simulink model "tests"  (R2024b)
settings: Solver=VariableStepAuto  StartTime=0.0  StopTime=1  RelTol=1e-3  AbsTol=1e-3  EnableMultiTasking=on
values from neighbouring files (symbols this model uses):
  m = obj.Br *obj.volume / obj.mu    [External_Magnet2.m]
  N = gridSizes(k)    [Test.m]
  Params = Sim_Param_Setup    [Sim_Open.m]
undefined symbols (not defined in the file or in its folder): X, Y, Z
libraries: sm_lib x88, vrlib x72, nesl_utility x52, matrix_library x46, sharedtransform x6
(part 2 of 5)

== system tests/Subsystem/Single_Arm/Plate_3 ==
  Pos_Plate6 : Inport
  M6 : Inport  Port=2
  Pos_Plate5 : Inport  Port=3
  M5 : Inport  Port=4
  Pos_Plate4 : Inport  Port=5
  M4 : Inport  Port=6
  Pos_Plate2 : Inport  Port=7
  M2 : Inport  Port=8
  Pos_Plate1 : Inport  Port=9
  M1 : Inport  Port=10
  Source_Pos : Inport  Port=11
  Source_Moment : Inport  Port=12
  Brick Solid : sm_lib/Body Elements/Brick Solid  BrickDimensions=[Params.LinkWidth Params.LinkThickness Params.LinkLength]  BrickDimensionsUnits=m  ExportEntireGeometry=off  InertiaType=CalculateFromGeometry  BasedOnType=Density  Density=1000  DensityUnits=kg/m^3  Mass=1  MassUnits=kg  CenterOfMass=[0 0 0]  CenterOfMassUnits=m  MomentsOfInertia=[1 1 1]  MomentsOfInertiaUnits=kg*m^2  ProductsOfInertia=[0 0 0]  ProductsOfInertiaUnits=kg*m^2  GraphicType=FromGeometry  MarkerShape=Sphere  MarkerSize=10  GraphicVisPropType=SimpleVisualProperties  GraphicDiffuseColor=[0.5 0.5 0.5]  GraphicOpacity=0.5  GraphicSpecularColor=[0.5 0.5 0.5 1.0]  GraphicAmbientColor=[0.15 0.15 0.15 1.0]  GraphicEmissiveColor=[0.0 0.0 0.0 1.0]  GraphicShininess=75  DoExposeReferenceFrame=on  SerializedFrames=<Frames><Frame><Id>Frame1</Id><Value><Name>F1</Name><Origin><Source>GeometricFeature</Source><FeatureName>-x -y curve</FeatureName></Origin><PrimaryAxis><DefinedDirection>+Z</DefinedDirection><Source>ReferenceFrame</Source><SourceDirection>+Z</SourceDirection><FeatureName></FeatureName></PrimaryAxis><SecondaryAxis><DefinedDirection>+X</DefinedDirection><Source>ReferenceFrame</Source><SourceDirection>+X</SourceDirection><FeatureName></FeatureName></SecondaryAxis></Value></Frame><Frame><Id>Frame2</Id><Value><Name>F2</Name><Origin><Source>GeometricFeature</Source><FeatureName>+x -y curve</FeatureName></Origin><PrimaryAxis><DefinedDirection>+Z</DefinedDirection><Source>ReferenceFrame</Source><SourceDirection>+Z</SourceDirection><FeatureName></FeatureName></PrimaryAxis><SecondaryAxis><DefinedDirection>+X</DefinedDirection><Source>ReferenceFrame</Source><SourceDirection>+X</SourceDirection><FeatureName></FeatureName></SecondaryAxis></Value></Frame></Frames>
  Constant : Constant  Value=[1; 0; 0]  VectorParams1D=off
  "Dipole Moment Angle Rot(z, theta)" : sm_lib/Frames and Transforms/Rigid Transform  RotationMethod=StandardAxis  FollAlignAxisA=+X  BaseAlignAxisA=+Y  FollAlignAxisB=+Y  BaseAlignAxisB=+Z  RotationStandardAxis=+Z  RotationAngle=Params.Link_Magnetization_Angle(3)  RotationAngleUnits=deg  RotationArbitraryAxis=[0 0 1]  RotationSequenceAxes=FollowerAxes  RotationSequence=XYX  RotationSequenceAngles=[0 0 0]  RotationSequenceAnglesUnits=deg  RotationMatrix=[1 0 0;0 1 0;0 0 1]  Quaternion=[1 0 0 0]  TranslationMethod=None  TranslationCartesianOffset=[0 0 0]  TranslationCartesianOffsetUnits=m  TranslationStandardAxis=+Z  TranslationStandardOffset=0  TranslationStandardOffsetUnits=m  TranslationROffset=0  TranslationROffsetUnits=m  TranslationThetaOffset=0  TranslationThetaOffsetUnits=deg  TranslationZOffset=0  TranslationZOffsetUnits=m
  External Force and Torque : sm_lib/Forces and Torques/External Force and Torque  EnableForceX=off  EnableForceY=off  EnableForceZ=off  EnableForce=on  ForceResolutionFrame=AttachedFrame  EnableTorqueX=off  EnableTorqueY=off  EnableTorqueZ=off  EnableTorque=on  TorqueResolutionFrame=AttachedFrame
  External Force and Torque1 : sm_lib/Forces and Torques/External Force and Torque  EnableForceX=off  EnableForceY=off  EnableForceZ=off  EnableForce=on  ForceResolutionFrame=AttachedFrame  EnableTorqueX=off  EnableTorqueY=off  EnableTorqueZ=off  EnableTorque=on  TorqueResolutionFrame=AttachedFrame
  Gain : Gain  Gain=Params.Link_Moment(3)
  PS-Simulink Converter : nesl_utility/PS-Simulink Converter  PhysicalDomain=network_engine_domain  SubClassName=ps_output  LeftPortType=input  RightPortType=output  PseudoPeriodic=off  Frequencies=[]  VectorFormat=inherit  Unit=inherit  AffineConversion=off
  PS-Simulink Converter2 : nesl_utility/PS-Simulink Converter  PhysicalDomain=network_engine_domain  SubClassName=ps_output  LeftPortType=input  RightPortType=output  PseudoPeriodic=off  Frequencies=[]  VectorFormat=inherit  Unit=inherit  AffineConversion=off
  Product : Product  Multiplication=Matrix(*)
  Revolved Solid : sm_lib/Body Elements/Revolved Solid  RevolutionCrossSection=[0 0; 1 0; 1 15; 2 15; 0 20]/10  RevolutionCrossSectionUnits=mm  RevolutionExtent=Full  RevolutionAngle=180  RevolutionAngleUnits=deg  ExportConvexHullGeometry=off  InertiaType=CalculateFromGeometry  BasedOnType=Density  Density=0  DensityUnits=kg/m^3  Mass=1  MassUnits=kg  CenterOfMass=[0 0 0]  CenterOfMassUnits=m  MomentsOfInertia=[1 1 1]  MomentsOfInertiaUnits=kg*m^2  ProductsOfInertia=[0 0 0]  ProductsOfInertiaUnits=kg*m^2  GraphicType=FromGeometry  MarkerShape=Sphere  MarkerSize=10  GraphicVisPropType=SimpleVisualProperties  GraphicDiffuseColor=[1 0 0]  GraphicOpacity=1  GraphicSpecularColor=[0.5 0.5 0.5 1.0]  GraphicAmbientColor=[0.15 0.15 0.15 1.0]  GraphicEmissiveColor=[0.0 0.0 0.0 1.0]  GraphicShininess=75  DoExposeReferenceFrame=on  SerializedFrames=<Frames/>
  Rigid Transform1 : sm_lib/Frames and Transforms/Rigid Transform  RotationMethod=StandardAxis  FollAlignAxisA=+X  BaseAlignAxisA=+Y  FollAlignAxisB=+Y  BaseAlignAxisB=+Z  RotationStandardAxis=+Y  RotationAngle=90  RotationAngleUnits=deg  RotationArbitraryAxis=[0 0 1]  RotationSequenceAxes=FollowerAxes  RotationSequence=XYX  RotationSequenceAngles=[0 0 0]  RotationSequenceAnglesUnits=deg  RotationMatrix=[1 0 0;0 1 0;0 0 1]  Quaternion=[1 0 0 0]  TranslationMethod=None  TranslationCartesianOffset=[0 0 0]  TranslationCartesianOffsetUnits=m  TranslationStandardAxis=+Z  TranslationStandardOffset=0  TranslationStandardOffsetUnits=m  TranslationROffset=0  TranslationROffsetUnits=m  TranslationThetaOffset=0  TranslationThetaOffsetUnits=deg  TranslationZOffset=0  TranslationZOffsetUnits=m
  Simulink-PS Converter{,1..3} (4 alike) : nesl_utility/Simulink-PS Converter  PhysicalDomain=network_engine_domain  SubClassName=ps_input  LeftPortType=input  RightPortType=output  PseudoPeriodic=off  Frequencies=[]  NoiseDistribution=none  NoiseParameters=[]  Unit=1  AffineConversion=off  FilteringAndDerivatives=provide  SimscapeFilterOrder=1  InputFilterTimeConstant=0.001  UdotUserProvided=0
  Subsystem : Subsystem
  Torques and Forces : Subsystem
      settings: PortSchema="{\"entries\":[{\"content\":{\"sides\":[{\"content\":{\"connectorIds\":[\"In1\",\"In2\",\"In3\",\"In4\",\"In5\",\"In6\",\"In7\",\"In8\",\"In9\",\"In10\",\"In11\",\"In12\"]},\"type\":\"ConnectorPlacement.EquallySpacedRectSide\",\"uuid\":\"5e9f7da2-fe68-4c7d-bff2-fdc8c7982441\"},{\"content\":{\"connectorIds\":[\"Out1\",\"Out2\"],\"side\":\"RIGHT\"},\"type\":\"ConnectorPlacement.EquallySpacedRectSide\",\"uuid\":\"36e5b3c2-6267-49a8-a0c4-2f3c1c270a99\"},{\"content\":{\"connectorIds\":[\"LConn1\"],\"side\":\"TOP\"},\"type\":\"ConnectorPlacement.EquallySpacedRectSide\",\"uuid\":\"f9d61316-4e06-4fe9-aa35-560b242a32a1\"}]},\"type\":\"ConnectorPlacement.EquallySpacedConnector\",\"uuid\":\"16298027-81d7-44cb-b7a6-bb815e806b74\"}],\"packageUris\":[\"http://schema.mathworks.com/mf0/Connector/R2020b\"],\"version\":\"1.0\"}"
  Transform Sensor : sm_lib/Frames and Transforms/Transform Sensor  MeasurementFrame=Base  RotationSequence=XYX  SenseAngle=off  SenseAxis=off  SenseQ=off  SenseR=on  SenseRotationSequence=off  SenseOmegaX=off  SenseOmegaY=off  SenseOmegaZ=off  SenseOmega=off  SenseQDot=off  SenseRDot=off  SenseRotationSequenceDot=off  SenseAlphaX=off  SenseAlphaY=off  SenseAlphaZ=off  SenseAlpha=off  SenseQDDot=off  SenseRDDot=off  SenseX=off  SenseY=off  SenseZ=off  SenseXYZ=on  SenseRad=off  SenseAzim=off  SenseDist=off  SenseInc=off  SenseXDot=off  SenseYDot=off  SenseZDot=off  SenseXYZDot=off  SenseRadDot=off  SenseAzimDot=off  SenseDistDot=off  SenseIncDot=off  SenseXDDot=off  SenseYDDot=off  SenseZDDot=off  SenseXYZDDot=off  SenseRadDDot=off  SenseAzimDDot=off  SenseDistDDot=off  SenseIncDDot=off
  World Frame : sm_lib/Frames and Transforms/World Frame
  Fixed one : PMIOPort  Side=Left
  base : PMIOPort  Port=2  Side=Right
  Pos_Plate3 : Outport
  M3 : Outport  Port=2
  wires:
  Gain/1 -> Product/2
  Constant/1 -> Gain/1
  Product/1 -> Torques and Forces/1(m_slave), Subsystem/1(Slave_Moment), M3/1
  PS-Simulink Converter2/1 -> Product/1
  PS-Simulink Converter/1 -> Pos_Plate3/1, Subsystem/2(Slave_Pos), Torques and Forces/2(Pos_Slave)
  M1/1 -> Torques and Forces/3(M1)
  Pos_Plate1/1 -> Torques and Forces/4(Pos_Plate1)
  M2/1 -> Torques and Forces/5(M2)
  Pos_Plate2/1 -> Torques and Forces/6(Pos_Plate2)
  M4/1 -> Torques and Forces/7(M4)
  Pos_Plate4/1 -> Torques and Forces/8(Pos_Plate4)
  M5/1 -> Torques and Forces/9(M5)
  Pos_Plate5/1 -> Torques and Forces/10(Pos_Plate5)
  M6/1 -> Torques and Forces/11(M6)
  Pos_Plate6/1 -> Torques and Forces/12(Pos_Plate6)
  Torques and Forces/1(Forces) -> Simulink-PS Converter/1
  Torques and Forces/2(Torques) -> Simulink-PS Converter1/1
  Source_Moment/1 -> Subsystem/3(Source_Moment)
  Source_Pos/1 -> Subsystem/4(Source_Pos)
  Subsystem/1(Source_Torque) -> Simulink-PS Converter3/1
  Subsystem/2(Source_Force) -> Simulink-PS Converter2/1
  connections:
  base/RConn1 -- Brick Solid/LConn1
  Brick Solid/LConn2 -- Fixed one/RConn1
  Rigid Transform1/LConn1 -- "Dipole Moment Angle Rot(z, theta)"/RConn1 -- Transform Sensor/RConn1
  Transform Sensor/RConn2 -- PS-Simulink Converter2/LConn1
  "Dipole Moment Angle Rot(z, theta)"/LConn1 -- Torques and Forces/LConn1 -- Brick Solid/RConn1 -- External Force and Torque/RConn1 -- External Force and Torque1/RConn1
  PS-Simulink Converter/LConn1 -- Transform Sensor/RConn3
  Rigid Transform1/RConn1 -- Revolved Solid/RConn1
  World Frame/RConn1 -- Transform Sensor/LConn1
  Simulink-PS Converter/RConn1 -- External Force and Torque/LConn1
  External Force and Torque/LConn2 -- Simulink-PS Converter1/RConn1
  External Force and Torque1/LConn1 -- Simulink-PS Converter2/RConn1
  Simulink-PS Converter3/RConn1 -- External Force and Torque1/LConn2

== system tests/Subsystem/Single_Arm/Plate_4 ==
  Pos_Plate6 : Inport
  M6 : Inport  Port=2
  Pos_Plate5 : Inport  Port=3
  M5 : Inport  Port=4
  Pos_Plate3 : Inport  Port=5
  M3 : Inport  Port=6
  Pos_Plate2 : Inport  Port=7
  M2 : Inport  Port=8
  Pos_Plate1 : Inport  Port=9
  M1 : Inport  Port=10
  Source_Pos : Inport  Port=11
  Source_Moment : Inport  Port=12
  Brick Solid : sm_lib/Body Elements/Brick Solid  BrickDimensions=[Params.LinkWidth Params.LinkThickness Params.LinkLength]  BrickDimensionsUnits=m  ExportEntireGeometry=off  InertiaType=CalculateFromGeometry  BasedOnType=Density  Density=1000  DensityUnits=kg/m^3  Mass=1  MassUnits=kg  CenterOfMass=[0 0 0]  CenterOfMassUnits=m  MomentsOfInertia=[1 1 1]  MomentsOfInertiaUnits=kg*m^2  ProductsOfInertia=[0 0 0]  ProductsOfInertiaUnits=kg*m^2  GraphicType=FromGeometry  MarkerShape=Sphere  MarkerSize=10  GraphicVisPropType=SimpleVisualProperties  GraphicDiffuseColor=[0.5 0.5 0.5]  GraphicOpacity=0.5  GraphicSpecularColor=[0.5 0.5 0.5 1.0]  GraphicAmbientColor=[0.15 0.15 0.15 1.0]  GraphicEmissiveColor=[0.0 0.0 0.0 1.0]  GraphicShininess=75  DoExposeReferenceFrame=on  SerializedFrames=<Frames><Frame><Id>Frame1</Id><Value><Name>F1</Name><Origin><Source>GeometricFeature</Source><FeatureName>-x -y curve</FeatureName></Origin><PrimaryAxis><DefinedDirection>+Z</DefinedDirection><Source>ReferenceFrame</Source><SourceDirection>+Z</SourceDirection><FeatureName></FeatureName></PrimaryAxis><SecondaryAxis><DefinedDirection>+X</DefinedDirection><Source>ReferenceFrame</Source><SourceDirection>+X</SourceDirection><FeatureName></FeatureName></SecondaryAxis></Value></Frame><Frame><Id>Frame2</Id><Value><Name>F2</Name><Origin><Source>GeometricFeature</Source><FeatureName>+x -y curve</FeatureName></Origin><PrimaryAxis><DefinedDirection>+Z</DefinedDirection><Source>ReferenceFrame</Source><SourceDirection>+Z</SourceDirection><FeatureName></FeatureName></PrimaryAxis><SecondaryAxis><DefinedDirection>+X</DefinedDirection><Source>ReferenceFrame</Source><SourceDirection>+X</SourceDirection><FeatureName></FeatureName></SecondaryAxis></Value></Frame></Frames>
  Constant : Constant  Value=[1; 0; 0]  VectorParams1D=off
  "Dipole Moment Angle Rot(z, theta)" : sm_lib/Frames and Transforms/Rigid Transform  RotationMethod=StandardAxis  FollAlignAxisA=+X  BaseAlignAxisA=+Y  FollAlignAxisB=+Y  BaseAlignAxisB=+Z  RotationStandardAxis=+Z  RotationAngle=Params.Link_Magnetization_Angle(4)  RotationAngleUnits=deg  RotationArbitraryAxis=[0 0 1]  RotationSequenceAxes=FollowerAxes  RotationSequence=XYX  RotationSequenceAngles=[0 0 0]  RotationSequenceAnglesUnits=deg  RotationMatrix=[1 0 0;0 1 0;0 0 1]  Quaternion=[1 0 0 0]  TranslationMethod=None  TranslationCartesianOffset=[0 0 0]  TranslationCartesianOffsetUnits=m  TranslationStandardAxis=+Z  TranslationStandardOffset=0  TranslationStandardOffsetUnits=m  TranslationROffset=0  TranslationROffsetUnits=m  TranslationThetaOffset=0  TranslationThetaOffsetUnits=deg  TranslationZOffset=0  TranslationZOffsetUnits=m
  External Force and Torque : sm_lib/Forces and Torques/External Force and Torque  EnableForceX=off  EnableForceY=off  EnableForceZ=off  EnableForce=on  ForceResolutionFrame=AttachedFrame  EnableTorqueX=off  EnableTorqueY=off  EnableTorqueZ=off  EnableTorque=on  TorqueResolutionFrame=AttachedFrame
  External Force and Torque1 : sm_lib/Forces and Torques/External Force and Torque  EnableForceX=off  EnableForceY=off  EnableForceZ=off  EnableForce=on  ForceResolutionFrame=AttachedFrame  EnableTorqueX=off  EnableTorqueY=off  EnableTorqueZ=off  EnableTorque=on  TorqueResolutionFrame=AttachedFrame
  Gain : Gain  Gain=Params.Link_Moment(4)
  PS-Simulink Converter : nesl_utility/PS-Simulink Converter  PhysicalDomain=network_engine_domain  SubClassName=ps_output  LeftPortType=input  RightPortType=output  PseudoPeriodic=off  Frequencies=[]  VectorFormat=inherit  Unit=inherit  AffineConversion=off
  PS-Simulink Converter2 : nesl_utility/PS-Simulink Converter  PhysicalDomain=network_engine_domain  SubClassName=ps_output  LeftPortType=input  RightPortType=output  PseudoPeriodic=off  Frequencies=[]  VectorFormat=inherit  Unit=inherit  AffineConversion=off
  Product : Product  Multiplication=Matrix(*)
  Revolved Solid : sm_lib/Body Elements/Revolved Solid  RevolutionCrossSection=[0 0; 1 0; 1 15; 2 15; 0 20]/10  RevolutionCrossSectionUnits=mm  RevolutionExtent=Full  RevolutionAngle=180  RevolutionAngleUnits=deg  ExportConvexHullGeometry=off  InertiaType=CalculateFromGeometry  BasedOnType=Density  Density=0  DensityUnits=kg/m^3  Mass=1  MassUnits=kg  CenterOfMass=[0 0 0]  CenterOfMassUnits=m  MomentsOfInertia=[1 1 1]  MomentsOfInertiaUnits=kg*m^2  ProductsOfInertia=[0 0 0]  ProductsOfInertiaUnits=kg*m^2  GraphicType=FromGeometry  MarkerShape=Sphere  MarkerSize=10  GraphicVisPropType=SimpleVisualProperties  GraphicDiffuseColor=[1 0 0]  GraphicOpacity=1  GraphicSpecularColor=[0.5 0.5 0.5 1.0]  GraphicAmbientColor=[0.15 0.15 0.15 1.0]  GraphicEmissiveColor=[0.0 0.0 0.0 1.0]  GraphicShininess=75  DoExposeReferenceFrame=on  SerializedFrames=<Frames/>
  Rigid Transform1 : sm_lib/Frames and Transforms/Rigid Transform  RotationMethod=StandardAxis  FollAlignAxisA=+X  BaseAlignAxisA=+Y  FollAlignAxisB=+Y  BaseAlignAxisB=+Z  RotationStandardAxis=+Y  RotationAngle=90  RotationAngleUnits=deg  RotationArbitraryAxis=[0 0 1]  RotationSequenceAxes=FollowerAxes  RotationSequence=XYX  RotationSequenceAngles=[0 0 0]  RotationSequenceAnglesUnits=deg  RotationMatrix=[1 0 0;0 1 0;0 0 1]  Quaternion=[1 0 0 0]  TranslationMethod=None  TranslationCartesianOffset=[0 0 0]  TranslationCartesianOffsetUnits=m  TranslationStandardAxis=+Z  TranslationStandardOffset=0  TranslationStandardOffsetUnits=m  TranslationROffset=0  TranslationROffsetUnits=m  TranslationThetaOffset=0  TranslationThetaOffsetUnits=deg  TranslationZOffset=0  TranslationZOffsetUnits=m
  Simulink-PS Converter{,1..3} (4 alike) : nesl_utility/Simulink-PS Converter  PhysicalDomain=network_engine_domain  SubClassName=ps_input  LeftPortType=input  RightPortType=output  PseudoPeriodic=off  Frequencies=[]  NoiseDistribution=none  NoiseParameters=[]  Unit=1  AffineConversion=off  FilteringAndDerivatives=provide  SimscapeFilterOrder=1  InputFilterTimeConstant=0.001  UdotUserProvided=0
  Subsystem : Subsystem
  Torques and Forces : Subsystem
      settings: PortSchema="{\"entries\":[{\"content\":{\"sides\":[{\"content\":{\"connectorIds\":[\"In1\",\"In2\",\"In3\",\"In4\",\"In5\",\"In6\",\"In7\",\"In8\",\"In9\",\"In10\",\"In11\",\"In12\"]},\"type\":\"ConnectorPlacement.EquallySpacedRectSide\",\"uuid\":\"5e9f7da2-fe68-4c7d-bff2-fdc8c7982441\"},{\"content\":{\"connectorIds\":[\"Out1\",\"Out2\"],\"side\":\"RIGHT\"},\"type\":\"ConnectorPlacement.EquallySpacedRectSide\",\"uuid\":\"36e5b3c2-6267-49a8-a0c4-2f3c1c270a99\"},{\"content\":{\"connectorIds\":[\"LConn1\"],\"side\":\"TOP\"},\"type\":\"ConnectorPlacement.EquallySpacedRectSide\",\"uuid\":\"f9d61316-4e06-4fe9-aa35-560b242a32a1\"}]},\"type\":\"ConnectorPlacement.EquallySpacedConnector\",\"uuid\":\"16298027-81d7-44cb-b7a6-bb815e806b74\"}],\"packageUris\":[\"http://schema.mathworks.com/mf0/Connector/R2020b\"],\"version\":\"1.0\"}"
  Transform Sensor : sm_lib/Frames and Transforms/Transform Sensor  MeasurementFrame=Base  RotationSequence=XYX  SenseAngle=off  SenseAxis=off  SenseQ=off  SenseR=on  SenseRotationSequence=off  SenseOmegaX=off  SenseOmegaY=off  SenseOmegaZ=off  SenseOmega=off  SenseQDot=off  SenseRDot=off  SenseRotationSequenceDot=off  SenseAlphaX=off  SenseAlphaY=off  SenseAlphaZ=off  SenseAlpha=off  SenseQDDot=off  SenseRDDot=off  SenseX=off  SenseY=off  SenseZ=off  SenseXYZ=on  SenseRad=off  SenseAzim=off  SenseDist=off  SenseInc=off  SenseXDot=off  SenseYDot=off  SenseZDot=off  SenseXYZDot=off  SenseRadDot=off  SenseAzimDot=off  SenseDistDot=off  SenseIncDot=off  SenseXDDot=off  SenseYDDot=off  SenseZDDot=off  SenseXYZDDot=off  SenseRadDDot=off  SenseAzimDDot=off  SenseDistDDot=off  SenseIncDDot=off
  World Frame : sm_lib/Frames and Transforms/World Frame
  Fixed one : PMIOPort  Side=Left
  base : PMIOPort  Port=2  Side=Right
  Pos_Plate4 : Outport
  M4 : Outport  Port=2
  wires:
  PS-Simulink Converter/1 -> Subsystem/2(Slave_Pos), Torques and Forces/2(Pos_Slave), Pos_Plate4/1
  Product/1 -> Torques and Forces/1(m_slave), Subsystem/1(Slave_Moment), M4/1
  Gain/1 -> Product/2
  Constant/1 -> Gain/1
  PS-Simulink Converter2/1 -> Product/1
  M1/1 -> Torques and Forces/3(M1)
  Pos_Plate1/1 -> Torques and Forces/4(Pos_Plate1)
  M2/1 -> Torques and Forces/5(M2)
  Pos_Plate2/1 -> Torques and Forces/6(Pos_Plate2)
  M3/1 -> Torques and Forces/7(M3)
  Pos_Plate3/1 -> Torques and Forces/8(Pos_Plate3)
  M5/1 -> Torques and Forces/9(M5)
  Pos_Plate5/1 -> Torques and Forces/10(Pos_Plate5)
  M6/1 -> Torques and Forces/11(M6)
  Pos_Plate6/1 -> Torques and Forces/12(Pos_Plate6)
  Torques and Forces/1(Forces) -> Simulink-PS Converter/1
  Torques and Forces/2(Torques) -> Simulink-PS Converter1/1
  Source_Moment/1 -> Subsystem/3(Source_Moment)
  Source_Pos/1 -> Subsystem/4(Source_Pos)
  Subsystem/1(Source_Torque) -> Simulink-PS Converter3/1
  Subsystem/2(Source_Force) -> Simulink-PS Converter2/1
  connections:
  base/RConn1 -- Brick Solid/LConn1
  Brick Solid/LConn2 -- Fixed one/RConn1
  Rigid Transform1/LConn1 -- "Dipole Moment Angle Rot(z, theta)"/RConn1 -- Transform Sensor/RConn1
  World Frame/RConn1 -- Transform Sensor/LConn1
  Rigid Transform1/RConn1 -- Revolved Solid/RConn1
  PS-Simulink Converter/LConn1 -- Transform Sensor/RConn3
  Brick Solid/RConn1 -- Torques and Forces/LConn1 -- External Force and Torque/RConn1 -- External Force and Torque1/RConn1 -- "Dipole Moment Angle Rot(z, theta)"/LConn1
  Transform Sensor/RConn2 -- PS-Simulink Converter2/LConn1
  External Force and Torque/LConn2 -- Simulink-PS Converter1/RConn1
  Simulink-PS Converter/RConn1 -- External Force and Torque/LConn1
  External Force and Torque1/LConn1 -- Simulink-PS Converter2/RConn1
  Simulink-PS Converter3/RConn1 -- External Force and Torque1/LConn2

== system tests/Subsystem/Single_Arm/Plate_5 ==
  Pos_Plate6 : Inport
  M6 : Inport  Port=2
  Pos_Plate4 : Inport  Port=3
  M4 : Inport  Port=4
  Pos_Plate3 : Inport  Port=5
  M3 : Inport  Port=6
  Pos_Plate2 : Inport  Port=7
  M2 : Inport  Port=8
  Pos_Plate1 : Inport  Port=9
  M1 : Inport  Port=10
  Source_Pos : Inport  Port=11
  Source_Moment : Inport  Port=12
  Brick Solid : sm_lib/Body Elements/Brick Solid  BrickDimensions=[Params.LinkWidth Params.LinkThickness Params.LinkLength]  BrickDimensionsUnits=m  ExportEntireGeometry=off  InertiaType=CalculateFromGeometry  BasedOnType=Density  Density=1000  DensityUnits=kg/m^3  Mass=1  MassUnits=kg  CenterOfMass=[0 0 0]  CenterOfMassUnits=m  MomentsOfInertia=[1 1 1]  MomentsOfInertiaUnits=kg*m^2  ProductsOfInertia=[0 0 0]  ProductsOfInertiaUnits=kg*m^2  GraphicType=FromGeometry  MarkerShape=Sphere  MarkerSize=10  GraphicVisPropType=SimpleVisualProperties  GraphicDiffuseColor=[0.5 0.5 0.5]  GraphicOpacity=0.5  GraphicSpecularColor=[0.5 0.5 0.5 1.0]  GraphicAmbientColor=[0.15 0.15 0.15 1.0]  GraphicEmissiveColor=[0.0 0.0 0.0 1.0]  GraphicShininess=75  DoExposeReferenceFrame=on  SerializedFrames=<Frames><Frame><Id>Frame1</Id><Value><Name>F1</Name><Origin><Source>GeometricFeature</Source><FeatureName>-x -y curve</FeatureName></Origin><PrimaryAxis><DefinedDirection>+Z</DefinedDirection><Source>ReferenceFrame</Source><SourceDirection>+Z</SourceDirection><FeatureName></FeatureName></PrimaryAxis><SecondaryAxis><DefinedDirection>+X</DefinedDirection><Source>ReferenceFrame</Source><SourceDirection>+X</SourceDirection><FeatureName></FeatureName></SecondaryAxis></Value></Frame><Frame><Id>Frame2</Id><Value><Name>F2</Name><Origin><Source>GeometricFeature</Source><FeatureName>+x -y curve</FeatureName></Origin><PrimaryAxis><DefinedDirection>+Z</DefinedDirection><Source>ReferenceFrame</Source><SourceDirection>+Z</SourceDirection><FeatureName></FeatureName></PrimaryAxis><SecondaryAxis><DefinedDirection>+X</DefinedDirection><Source>ReferenceFrame</Source><SourceDirection>+X</SourceDirection><FeatureName></FeatureName></SecondaryAxis></Value></Frame></Frames>
  Constant : Constant  Value=[1; 0; 0]  VectorParams1D=off
  "Dipole Moment Angle Rot(z, theta)" : sm_lib/Frames and Transforms/Rigid Transform  RotationMethod=StandardAxis  FollAlignAxisA=+X  BaseAlignAxisA=+Y  FollAlignAxisB=+Y  BaseAlignAxisB=+Z  RotationStandardAxis=+Z  RotationAngle=Params.Link_Magnetization_Angle(5)  RotationAngleUnits=deg  RotationArbitraryAxis=[0 0 1]  RotationSequenceAxes=FollowerAxes  RotationSequence=XYX  RotationSequenceAngles=[0 0 0]  RotationSequenceAnglesUnits=deg  RotationMatrix=[1 0 0;0 1 0;0 0 1]  Quaternion=[1 0 0 0]  TranslationMethod=None  TranslationCartesianOffset=[0 0 0]  TranslationCartesianOffsetUnits=m  TranslationStandardAxis=+Z  TranslationStandardOffset=0  TranslationStandardOffsetUnits=m  TranslationROffset=0  TranslationROffsetUnits=m  TranslationThetaOffset=0  TranslationThetaOffsetUnits=deg  TranslationZOffset=0  TranslationZOffsetUnits=m
  External Force and Torque : sm_lib/Forces and Torques/External Force and Torque  EnableForceX=off  EnableForceY=off  EnableForceZ=off  EnableForce=on  ForceResolutionFrame=AttachedFrame  EnableTorqueX=off  EnableTorqueY=off  EnableTorqueZ=off  EnableTorque=on  TorqueResolutionFrame=AttachedFrame
  External Force and Torque1 : sm_lib/Forces and Torques/External Force and Torque  EnableForceX=off  EnableForceY=off  EnableForceZ=off  EnableForce=on  ForceResolutionFrame=AttachedFrame  EnableTorqueX=off  EnableTorqueY=off  EnableTorqueZ=off  EnableTorque=on  TorqueResolutionFrame=AttachedFrame
  Gain : Gain  Gain=Params.Link_Moment(5)
  PS-Simulink Converter : nesl_utility/PS-Simulink Converter  PhysicalDomain=network_engine_domain  SubClassName=ps_output  LeftPortType=input  RightPortType=output  PseudoPeriodic=off  Frequencies=[]  VectorFormat=inherit  Unit=inherit  AffineConversion=off
  PS-Simulink Converter2 : nesl_utility/PS-Simulink Converter  PhysicalDomain=network_engine_domain  SubClassName=ps_output  LeftPortType=input  RightPortType=output  PseudoPeriodic=off  Frequencies=[]  VectorFormat=inherit  Unit=inherit  AffineConversion=off
  Product : Product  Multiplication=Matrix(*)
  Revolved Solid : sm_lib/Body Elements/Revolved Solid  RevolutionCrossSection=[0 0; 1 0; 1 15; 2 15; 0 20]/10  RevolutionCrossSectionUnits=mm  RevolutionExtent=Full  RevolutionAngle=180  RevolutionAngleUnits=deg  ExportConvexHullGeometry=off  InertiaType=CalculateFromGeometry  BasedOnType=Density  Density=0  DensityUnits=kg/m^3  Mass=1  MassUnits=kg  CenterOfMass=[0 0 0]  CenterOfMassUnits=m  MomentsOfInertia=[1 1 1]  MomentsOfInertiaUnits=kg*m^2  ProductsOfInertia=[0 0 0]  ProductsOfInertiaUnits=kg*m^2  GraphicType=FromGeometry  MarkerShape=Sphere  MarkerSize=10  GraphicVisPropType=SimpleVisualProperties  GraphicDiffuseColor=[1 0 0]  GraphicOpacity=1  GraphicSpecularColor=[0.5 0.5 0.5 1.0]  GraphicAmbientColor=[0.15 0.15 0.15 1.0]  GraphicEmissiveColor=[0.0 0.0 0.0 1.0]  GraphicShininess=75  DoExposeReferenceFrame=on  SerializedFrames=<Frames/>
  Rigid Transform1 : sm_lib/Frames and Transforms/Rigid Transform  RotationMethod=StandardAxis  FollAlignAxisA=+X  BaseAlignAxisA=+Y  FollAlignAxisB=+Y  BaseAlignAxisB=+Z  RotationStandardAxis=+Y  RotationAngle=90  RotationAngleUnits=deg  RotationArbitraryAxis=[0 0 1]  RotationSequenceAxes=FollowerAxes  RotationSequence=XYX  RotationSequenceAngles=[0 0 0]  RotationSequenceAnglesUnits=deg  RotationMatrix=[1 0 0;0 1 0;0 0 1]  Quaternion=[1 0 0 0]  TranslationMethod=None  TranslationCartesianOffset=[0 0 0]  TranslationCartesianOffsetUnits=m  TranslationStandardAxis=+Z  TranslationStandardOffset=0  TranslationStandardOffsetUnits=m  TranslationROffset=0  TranslationROffsetUnits=m  TranslationThetaOffset=0  TranslationThetaOffsetUnits=deg  TranslationZOffset=0  TranslationZOffsetUnits=m
  Simulink-PS Converter{,1..3} (4 alike) : nesl_utility/Simulink-PS Converter  PhysicalDomain=network_engine_domain  SubClassName=ps_input  LeftPortType=input  RightPortType=output  PseudoPeriodic=off  Frequencies=[]  NoiseDistribution=none  NoiseParameters=[]  Unit=1  AffineConversion=off  FilteringAndDerivatives=provide  SimscapeFilterOrder=1  InputFilterTimeConstant=0.001  UdotUserProvided=0
  Subsystem : Subsystem
  Torques and Forces : Subsystem
      settings: PortSchema="{\"entries\":[{\"content\":{\"sides\":[{\"content\":{\"connectorIds\":[\"In1\",\"In2\",\"In3\",\"In4\",\"In5\",\"In6\",\"In7\",\"In8\",\"In9\",\"In10\",\"In11\",\"In12\"]},\"type\":\"ConnectorPlacement.EquallySpacedRectSide\",\"uuid\":\"5e9f7da2-fe68-4c7d-bff2-fdc8c7982441\"},{\"content\":{\"connectorIds\":[\"Out1\",\"Out2\"],\"side\":\"RIGHT\"},\"type\":\"ConnectorPlacement.EquallySpacedRectSide\",\"uuid\":\"36e5b3c2-6267-49a8-a0c4-2f3c1c270a99\"},{\"content\":{\"connectorIds\":[\"LConn1\"],\"side\":\"TOP\"},\"type\":\"ConnectorPlacement.EquallySpacedRectSide\",\"uuid\":\"f9d61316-4e06-4fe9-aa35-560b242a32a1\"}]},\"type\":\"ConnectorPlacement.EquallySpacedConnector\",\"uuid\":\"16298027-81d7-44cb-b7a6-bb815e806b74\"}],\"packageUris\":[\"http://schema.mathworks.com/mf0/Connector/R2020b\"],\"version\":\"1.0\"}"
  Transform Sensor : sm_lib/Frames and Transforms/Transform Sensor  MeasurementFrame=Base  RotationSequence=XYX  SenseAngle=off  SenseAxis=off  SenseQ=off  SenseR=on  SenseRotationSequence=off  SenseOmegaX=off  SenseOmegaY=off  SenseOmegaZ=off  SenseOmega=off  SenseQDot=off  SenseRDot=off  SenseRotationSequenceDot=off  SenseAlphaX=off  SenseAlphaY=off  SenseAlphaZ=off  SenseAlpha=off  SenseQDDot=off  SenseRDDot=off  SenseX=off  SenseY=off  SenseZ=off  SenseXYZ=on  SenseRad=off  SenseAzim=off  SenseDist=off  SenseInc=off  SenseXDot=off  SenseYDot=off  SenseZDot=off  SenseXYZDot=off  SenseRadDot=off  SenseAzimDot=off  SenseDistDot=off  SenseIncDot=off  SenseXDDot=off  SenseYDDot=off  SenseZDDot=off  SenseXYZDDot=off  SenseRadDDot=off  SenseAzimDDot=off  SenseDistDDot=off  SenseIncDDot=off
  World Frame : sm_lib/Frames and Transforms/World Frame
  Fixed one : PMIOPort  Side=Left
  base : PMIOPort  Port=2  Side=Right
  Pos_Plate5 : Outport
  M5 : Outport  Port=2
  wires:
  PS-Simulink Converter/1 -> Subsystem/2(Slave_Pos), Torques and Forces/2(Pos_Slave), Pos_Plate5/1
  Product/1 -> Torques and Forces/1(m_slave), Subsystem/1(Slave_Moment), M5/1
  Gain/1 -> Product/2
  Constant/1 -> Gain/1
  PS-Simulink Converter2/1 -> Product/1
  M1/1 -> Torques and Forces/3(M1)
  Pos_Plate1/1 -> Torques and Forces/4(Pos_Plate1)
  M2/1 -> Torques and Forces/5(M2)
  Pos_Plate2/1 -> Torques and Forces/6(Pos_Plate2)
  M3/1 -> Torques and Forces/7(M3)
  Pos_Plate3/1 -> Torques and Forces/8(Pos_Plate3)
  M4/1 -> Torques and Forces/9(M4)
  Pos_Plate4/1 -> Torques and Forces/10(Pos_Plate4)
  M6/1 -> Torques and Forces/11(M6)
  Pos_Plate6/1 -> Torques and Forces/12(Pos_Plate6)
  Torques and Forces/1(Forces) -> Simulink-PS Converter/1
  Torques and Forces/2(Torques) -> Simulink-PS Converter1/1
  Source_Moment/1 -> Subsystem/3(Source_Moment)
  Source_Pos/1 -> Subsystem/4(Source_Pos)
  Subsystem/1(Source_Torque) -> Simulink-PS Converter3/1
  Subsystem/2(Source_Force) -> Simulink-PS Converter2/1
  connections:
  base/RConn1 -- Brick Solid/LConn1
  Brick Solid/LConn2 -- Fixed one/RConn1
  Rigid Transform1/LConn1 -- "Dipole Moment Angle Rot(z, theta)"/RConn1 -- Transform Sensor/RConn1
  World Frame/RConn1 -- Transform Sensor/LConn1
  Rigid Transform1/RConn1 -- Revolved Solid/RConn1
  PS-Simulink Converter/LConn1 -- Transform Sensor/RConn3
  Brick Solid/RConn1 -- External Force and Torque1/RConn1 -- "Dipole Moment Angle Rot(z, theta)"/LConn1 -- External Force and Torque/RConn1 -- Torques and Forces/LConn1
  Transform Sensor/RConn2 -- PS-Simulink Converter2/LConn1
  External Force and Torque/LConn2 -- Simulink-PS Converter1/RConn1
  Simulink-PS Converter/RConn1 -- External Force and Torque/LConn1
  External Force and Torque1/LConn1 -- Simulink-PS Converter2/RConn1
  Simulink-PS Converter3/RConn1 -- External Force and Torque1/LConn2

== system tests/Subsystem/Single_Arm/Plate_6 ==
  Pos_Plate5 : Inport
  M5 : Inport  Port=2
  Pos_Plate4 : Inport  Port=3
  M4 : Inport  Port=4
  Pos_Plate3 : Inport  Port=5
  M3 : Inport  Port=6
  Pos_Plate2 : Inport  Port=7
  M2 : Inport  Port=8
  Pos_Plate1 : Inport  Port=9
  M1 : Inport  Port=10
  Source_Pos : Inport  Port=11
  Source_Moment : Inport  Port=12
  Brick Solid : sm_lib/Body Elements/Brick Solid  BrickDimensions=[Params.LinkWidth Params.LinkThickness Params.LinkLength]  BrickDimensionsUnits=m  ExportEntireGeometry=off  InertiaType=CalculateFromGeometry  BasedOnType=Density  Density=1000  DensityUnits=kg/m^3  Mass=1  MassUnits=kg  CenterOfMass=[0 0 0]  CenterOfMassUnits=m  MomentsOfInertia=[1 1 1]  MomentsOfInertiaUnits=kg*m^2  ProductsOfInertia=[0 0 0]  ProductsOfInertiaUnits=kg*m^2  GraphicType=FromGeometry  MarkerShape=Sphere  MarkerSize=10  GraphicVisPropType=SimpleVisualProperties  GraphicDiffuseColor=[0.5 0.5 0.5]  GraphicOpacity=0.5  GraphicSpecularColor=[0.5 0.5 0.5 1.0]  GraphicAmbientColor=[0.15 0.15 0.15 1.0]  GraphicEmissiveColor=[0.0 0.0 0.0 1.0]  GraphicShininess=75  DoExposeReferenceFrame=on  SerializedFrames=<Frames><Frame><Id>Frame1</Id><Value><Name>F1</Name><Origin><Source>GeometricFeature</Source><FeatureName>-x -y curve</FeatureName></Origin><PrimaryAxis><DefinedDirection>+Z</DefinedDirection><Source>ReferenceFrame</Source><SourceDirection>+Z</SourceDirection><FeatureName></FeatureName></PrimaryAxis><SecondaryAxis><DefinedDirection>+X</DefinedDirection><Source>ReferenceFrame</Source><SourceDirection>+X</SourceDirection><FeatureName></FeatureName></SecondaryAxis></Value></Frame><Frame><Id>Frame2</Id><Value><Name>F2</Name><Origin><Source>GeometricFeature</Source><FeatureName>+x -y curve</FeatureName></Origin><PrimaryAxis><DefinedDirection>+Z</DefinedDirection><Source>ReferenceFrame</Source><SourceDirection>+Z</SourceDirection><FeatureName></FeatureName></PrimaryAxis><SecondaryAxis><DefinedDirection>+X</DefinedDirection><Source>ReferenceFrame</Source><SourceDirection>+X</SourceDirection><FeatureName></FeatureName></SecondaryAxis></Value></Frame></Frames>
  Constant : Constant  Value=[1; 0; 0]  VectorParams1D=off
  "Dipole Moment Angle Rot(z, theta)" : sm_lib/Frames and Transforms/Rigid Transform  RotationMethod=StandardAxis  FollAlignAxisA=+X  BaseAlignAxisA=+Y  FollAlignAxisB=+Y  BaseAlignAxisB=+Z  RotationStandardAxis=+Z  RotationAngle=Params.Link_Magnetization_Angle(6)  RotationAngleUnits=deg  RotationArbitraryAxis=[0 0 1]  RotationSequenceAxes=FollowerAxes  RotationSequence=XYX  RotationSequenceAngles=[0 0 0]  RotationSequenceAnglesUnits=deg  RotationMatrix=[1 0 0;0 1 0;0 0 1]  Quaternion=[1 0 0 0]  TranslationMethod=None  TranslationCartesianOffset=[0 0 0]  TranslationCartesianOffsetUnits=m  TranslationStandardAxis=+Z  TranslationStandardOffset=0  TranslationStandardOffsetUnits=m  TranslationROffset=0  TranslationROffsetUnits=m  TranslationThetaOffset=0  TranslationThetaOffsetUnits=deg  TranslationZOffset=0  TranslationZOffsetUnits=m
  External Force and Torque : sm_lib/Forces and Torques/External Force and Torque  EnableForceX=off  EnableForceY=off  EnableForceZ=off  EnableForce=on  ForceResolutionFrame=AttachedFrame  EnableTorqueX=off  EnableTorqueY=off  EnableTorqueZ=off  EnableTorque=on  TorqueResolutionFrame=AttachedFrame
  External Force and Torque1 : sm_lib/Forces and Torques/External Force and Torque  EnableForceX=off  EnableForceY=off  EnableForceZ=off  EnableForce=on  ForceResolutionFrame=AttachedFrame  EnableTorqueX=off  EnableTorqueY=off  EnableTorqueZ=off  EnableTorque=on  TorqueResolutionFrame=AttachedFrame
  Gain : Gain  Gain=Params.Link_Moment(6)
  PS-Simulink Converter : nesl_utility/PS-Simulink Converter  PhysicalDomain=network_engine_domain  SubClassName=ps_output  LeftPortType=input  RightPortType=output  PseudoPeriodic=off  Frequencies=[]  VectorFormat=inherit  Unit=inherit  AffineConversion=off
  PS-Simulink Converter2 : nesl_utility/PS-Simulink Converter  PhysicalDomain=network_engine_domain  SubClassName=ps_output  LeftPortType=input  RightPortType=output  PseudoPeriodic=off  Frequencies=[]  VectorFormat=inherit  Unit=inherit  AffineConversion=off
  Product : Product  Multiplication=Matrix(*)
  Revolved Solid : sm_lib/Body Elements/Revolved Solid  RevolutionCrossSection=[0 0; 1 0; 1 15; 2 15; 0 20]/10  RevolutionCrossSectionUnits=mm  RevolutionExtent=Full  RevolutionAngle=180  RevolutionAngleUnits=deg  ExportConvexHullGeometry=off  InertiaType=CalculateFromGeometry  BasedOnType=Density  Density=0  DensityUnits=kg/m^3  Mass=1  MassUnits=kg  CenterOfMass=[0 0 0]  CenterOfMassUnits=m  MomentsOfInertia=[1 1 1]  MomentsOfInertiaUnits=kg*m^2  ProductsOfInertia=[0 0 0]  ProductsOfInertiaUnits=kg*m^2  GraphicType=FromGeometry  MarkerShape=Sphere  MarkerSize=10  GraphicVisPropType=SimpleVisualProperties  GraphicDiffuseColor=[1 0 0]  GraphicOpacity=1  GraphicSpecularColor=[0.5 0.5 0.5 1.0]  GraphicAmbientColor=[0.15 0.15 0.15 1.0]  GraphicEmissiveColor=[0.0 0.0 0.0 1.0]  GraphicShininess=75  DoExposeReferenceFrame=on  SerializedFrames=<Frames/>
  Rigid Transform1 : sm_lib/Frames and Transforms/Rigid Transform  RotationMethod=StandardAxis  FollAlignAxisA=+X  BaseAlignAxisA=+Y  FollAlignAxisB=+Y  BaseAlignAxisB=+Z  RotationStandardAxis=+Y  RotationAngle=90  RotationAngleUnits=deg  RotationArbitraryAxis=[0 0 1]  RotationSequenceAxes=FollowerAxes  RotationSequence=XYX  RotationSequenceAngles=[0 0 0]  RotationSequenceAnglesUnits=deg  RotationMatrix=[1 0 0;0 1 0;0 0 1]  Quaternion=[1 0 0 0]  TranslationMethod=None  TranslationCartesianOffset=[0 0 0]  TranslationCartesianOffsetUnits=m  TranslationStandardAxis=+Z  TranslationStandardOffset=0  TranslationStandardOffsetUnits=m  TranslationROffset=0  TranslationROffsetUnits=m  TranslationThetaOffset=0  TranslationThetaOffsetUnits=deg  TranslationZOffset=0  TranslationZOffsetUnits=m
  Simulink-PS Converter{,1..3} (4 alike) : nesl_utility/Simulink-PS Converter  PhysicalDomain=network_engine_domain  SubClassName=ps_input  LeftPortType=input  RightPortType=output  PseudoPeriodic=off  Frequencies=[]  NoiseDistribution=none  NoiseParameters=[]  Unit=1  AffineConversion=off  FilteringAndDerivatives=provide  SimscapeFilterOrder=1  InputFilterTimeConstant=0.001  UdotUserProvided=0
  Subsystem : Subsystem
  Torques and Forces : Subsystem
      settings: PortSchema="{\"entries\":[{\"content\":{\"sides\":[{\"content\":{\"connectorIds\":[\"In1\",\"In2\",\"In3\",\"In4\",\"In5\",\"In6\",\"In7\",\"In8\",\"In9\",\"In10\",\"In11\",\"In12\"]},\"type\":\"ConnectorPlacement.EquallySpacedRectSide\",\"uuid\":\"ff28c452-50a3-45d4-b830-c141bf0d4924\"},{\"content\":{\"connectorIds\":[\"Out1\",\"Out2\"],\"side\":\"RIGHT\"},\"type\":\"ConnectorPlacement.EquallySpacedRectSide\",\"uuid\":\"4d65d73f-a147-470a-914d-b752947974df\"},{\"content\":{\"connectorIds\":[\"LConn1\"],\"side\":\"TOP\"},\"type\":\"ConnectorPlacement.EquallySpacedRectSide\",\"uuid\":\"638f3315-7fa0-4e2a-8069-7601753d6a25\"}]},\"type\":\"ConnectorPlacement.EquallySpacedConnector\",\"uuid\":\"2ec04731-f5c0-4183-a2fa-470eff73c2d9\"}],\"packageUris\":[\"http://schema.mathworks.com/mf0/Connector/R2020b\"],\"version\":\"1.0\"}"
  Transform Sensor : sm_lib/Frames and Transforms/Transform Sensor  MeasurementFrame=Base  RotationSequence=XYX  SenseAngle=off  SenseAxis=off  SenseQ=off  SenseR=on  SenseRotationSequence=off  SenseOmegaX=off  SenseOmegaY=off  SenseOmegaZ=off  SenseOmega=off  SenseQDot=off  SenseRDot=off  SenseRotationSequenceDot=off  SenseAlphaX=off  SenseAlphaY=off  SenseAlphaZ=off  SenseAlpha=off  SenseQDDot=off  SenseRDDot=off  SenseX=off  SenseY=off  SenseZ=off  SenseXYZ=on  SenseRad=off  SenseAzim=off  SenseDist=off  SenseInc=off  SenseXDot=off  SenseYDot=off  SenseZDot=off  SenseXYZDot=off  SenseRadDot=off  SenseAzimDot=off  SenseDistDot=off  SenseIncDot=off  SenseXDDot=off  SenseYDDot=off  SenseZDDot=off  SenseXYZDDot=off  SenseRadDDot=off  SenseAzimDDot=off  SenseDistDDot=off  SenseIncDDot=off
  World Frame : sm_lib/Frames and Transforms/World Frame
  Fixed one : PMIOPort  Side=Left
  base : PMIOPort  Port=2  Side=Right
  Pos_Plate6 : Outport
  M6 : Outport  Port=2
  wires:
  PS-Simulink Converter/1 -> Torques and Forces/2(Pos_Slave), Pos_Plate6/1, Subsystem/2(Slave_Pos)
  Product/1 -> Subsystem/1(Slave_Moment), Torques and Forces/1(m_slave), M6/1
  Gain/1 -> Product/2
  Constant/1 -> Gain/1
  PS-Simulink Converter2/1 -> Product/1
  M1/1 -> Torques and Forces/3(M1)
  Pos_Plate1/1 -> Torques and Forces/4(Pos_Plate1)
  M2/1 -> Torques and Forces/5(M2)
  Pos_Plate2/1 -> Torques and Forces/6(Pos_Plate2)
  M3/1 -> Torques and Forces/7(M3)
  Pos_Plate3/1 -> Torques and Forces/8(Pos_Plate3)
  M4/1 -> Torques and Forces/9(M4)
  Pos_Plate4/1 -> Torques and Forces/10(Pos_Plate4)
  M5/1 -> Torques and Forces/11(M5)
  Pos_Plate5/1 -> Torques and Forces/12(Pos_Plate5)
  Torques and Forces/1(Forces) -> Simulink-PS Converter/1
  Torques and Forces/2(Torques) -> Simulink-PS Converter1/1
  Source_Moment/1 -> Subsystem/3(Source_Moment)
  Source_Pos/1 -> Subsystem/4(Source_Pos)
  Subsystem/1(Source_Torque) -> Simulink-PS Converter3/1
  Subsystem/2(Source_Force) -> Simulink-PS Converter2/1
  connections:
  base/RConn1 -- Brick Solid/LConn1
  Brick Solid/LConn2 -- Fixed one/RConn1
  Rigid Transform1/LConn1 -- "Dipole Moment Angle Rot(z, theta)"/RConn1 -- Transform Sensor/RConn1
  World Frame/RConn1 -- Transform Sensor/LConn1
  Rigid Transform1/RConn1 -- Revolved Solid/RConn1
  PS-Simulink Converter/LConn1 -- Transform Sensor/RConn3
  Brick Solid/RConn1 -- External Force and Torque/RConn1 -- External Force and Torque1/RConn1 -- "Dipole Moment Angle Rot(z, theta)"/LConn1 -- Torques and Forces/LConn1
  Transform Sensor/RConn2 -- PS-Simulink Converter2/LConn1
  Simulink-PS Converter/RConn1 -- External Force and Torque/LConn1
  Simulink-PS Converter1/RConn1 -- External Force and Torque/LConn2
  External Force and Torque1/LConn1 -- Simulink-PS Converter2/RConn1
  Simulink-PS Converter3/RConn1 -- External Force and Torque1/LConn2

== system tests/Subsystem/Single_Arm/Plate_1/Subsystem ==
  Slave_Moment : Inport
  Slave_Pos : Inport  Port=2
  Source_Moment : Inport  Port=3
  Source_Pos : Inport  Port=4
  Add : Sum  Inputs=+-
  Add1 : Sum  Inputs=+-
  Add2 : Sum  Inputs=+-
  Add3 : Sum  Inputs=+++
  Constant : Constant  Value=-3
  Constant1 : Constant  Value=-4
  Cross Product : matrix_library/Cross Product
  Dot Product : DotProduct  OutDataTypeStr=Inherit: Inherit via internal rule
  Dot Product1 : DotProduct  OutDataTypeStr=Inherit: Inherit via internal rule
  Gain : Gain  Gain=4*pi*1e-7/(4*pi)
  Gain1 : Gain  Gain=3
  Gain2 : Gain  Gain=3*4*pi*1e-7/(4*pi)
  Gain3 : Gain  Gain=5
  IdentityMatrix : IdentityMatrix  OutputDimensions=3
  Matrix Multiply : Product  Multiplication=Matrix(*)
  Matrix Multiply1 : Product  Multiplication=Matrix(*)
  Normalize Vector : vrlib/Utilities/Normalize Vector  maxzero=0
  Normalize Vector1 : vrlib/Utilities/Normalize Vector  maxzero=0
  Power : Math  Operator=pow
  Power1 : Math  Operator=pow
  Product{,1..5} (6 alike) : Product
  Sqrt : Sqrt
  Sqrt1 : Sqrt
  Transpose : Math  Operator=transpose
  m dot m : DotProduct  OutDataTypeStr=Inherit: Inherit via internal rule
  r dot m_master : DotProduct  OutDataTypeStr=Inherit: Inherit via internal rule
  r dot m_slave : DotProduct  OutDataTypeStr=Inherit: Inherit via internal rule
  Source_Torque : Outport
  Source_Force : Outport  Port=2
  wires:
  Power/1 -> Gain/1
  Transpose/1 -> Matrix Multiply/2
  Gain1/1 -> Add/1
  Matrix Multiply/1 -> Gain1/1
  Sqrt/1 -> Power/1
  Gain/1 -> Product/2
  Dot Product/1 -> Sqrt/1
  Product/1 -> Cross Product/2
  Matrix Multiply1/1 -> Product/1
  Normalize Vector/1 -> Transpose/1, Matrix Multiply/1
  IdentityMatrix/1 -> Add/2
  Constant/1 -> Power/2
  Add/1 -> Matrix Multiply1/1
  Slave_Pos/1 -> Add1/1
  Source_Pos/1 -> Add1/2
  Cross Product/1 -> Source_Torque/1
  Slave_Moment/1 -> Cross Product/1, Product2/2, m dot m/1, r dot m_slave/2
  Normalize Vector1/1 -> r dot m_slave/1, r dot m_master/1, Product4/2
  Add3/1 -> Product5/2
  Gain2/1 -> Product5/1
  Product4/1 -> Add3/3
  Dot Product1/1 -> Sqrt1/1
  Gain3/1 -> Add2/2
  r dot m_master/1 -> Product3/2, Product2/1
  Source_Moment/1 -> Matrix Multiply1/2, m dot m/2, Product1/2, r dot m_master/2
  m dot m/1 -> Add2/1
  Power1/1 -> Gain2/1
  Sqrt1/1 -> Power1/1
  r dot m_slave/1 -> Product1/1, Product3/1
  Product2/1 -> Add3/2
  Constant1/1 -> Power1/2
  Add2/1 -> Product4/1
  Add1/1 -> Normalize Vector1/1, Dot Product1/2, Dot Product1/1, Dot Product/2, Dot Product/1, Normalize Vector/1
  Product3/1 -> Gain3/1
  Product1/1 -> Add3/1
  Product5/1 -> Source_Force/1

== system tests/Subsystem/Single_Arm/Plate_1/Torques and Forces ==
  m_slave : Inport
  Pos_Slave : Inport  Port=2
  M2 : Inport  Port=3
  Pos_Plate2 : Inport  Port=4
  M3 : Inport  Port=5
  Pos_Plate3 : Inport  Port=6
  M4 : Inport  Port=7
  Pos_Plate4 : Inport  Port=8
  M5 : Inport  Port=9
  Pos_Plate5 : Inport  Port=10
  M6 : Inport  Port=11
  Pos_Plate6 : Inport  Port=12
  Add{,1..4} (5 alike) : Sum  Inputs=+-
  Magnetic Forces : Subsystem
  Magnetic Torques : Subsystem
      settings: PortSchema="{\"entries\":[{\"content\":{\"sides\":[{\"content\":{\"connectorIds\":[\"In1\",\"In2\",\"In3\",\"In4\",\"In5\",\"In6\",\"In7\",\"In8\",\"In9\",\"In10\",\"In11\"]},\"type\":\"ConnectorPlacement.EquallySpacedRectSide\",\"uuid\":\"6f05c61b-28f4-4565-bbea-1be0fb93c6f0\"},{\"content\":{\"connectorIds\":[\"Out1\"],\"side\":\"RIGHT\"},\"type\":\"ConnectorPlacement.EquallySpacedRectSide\",\"uuid\":\"8634642c-fc93-4182-aaec-4f6aca47cd70\"},{\"content\":{\"connectorIds\":[\"LConn1\"],\"side\":\"TOP\"},\"type\":\"ConnectorPlacement.EquallySpacedRectSide\",\"uuid\":\"4c29c46f-a8de-4915-ac6e-9828579e7b84\"}]},\"type\":\"ConnectorPlacement.EquallySpacedConnector\",\"uuid\":\"3da81916-5d74-4352-a0fa-851a5433a86b\"}],\"packageUris\":[\"http://schema.mathworks.com/mf0/Connector/R2020b\"],\"version\":\"1.0\"}"
  brick reference : PMIOPort  Side=Left
  Forces : Outport
  Torques : Outport  Port=2
  wires:
  m_slave/1 -> Magnetic Forces/1(m_slave), Magnetic Torques/1(m_slave)
  Pos_Slave/1 -> Add4/1, Add3/1, Add2/1, Add1/1, Add/1
  Pos_Plate2/1 -> Add/2
  M2/1 -> Magnetic Torques/2(M2), Magnetic Forces/2(M2)
  Add/1 -> Magnetic Torques/7(r2), Magnetic Forces/7(r2)
  Pos_Plate6/1 -> Add4/2
  Pos_Plate5/1 -> Add3/2
  Pos_Plate4/1 -> Add2/2
  Pos_Plate3/1 -> Add1/2
  M3/1 -> Magnetic Forces/3(M3), Magnetic Torques/3(M3)
  Add1/1 -> Magnetic Torques/8(r3), Magnetic Forces/8(r3)
  M4/1 -> Magnetic Forces/4(M4), Magnetic Torques/4(M4)
  M5/1 -> Magnetic Forces/5(M5), Magnetic Torques/5(M5)
  M6/1 -> Magnetic Forces/6(M6), Magnetic Torques/6(M6)
  Add2/1 -> Magnetic Forces/9(r4), Magnetic Torques/9(r4)
  Add3/1 -> Magnetic Forces/10(r5), Magnetic Torques/10(r5)
  Add4/1 -> Magnetic Forces/11(r6), Magnetic Torques/11(r6)
  Magnetic Forces/1(Forces) -> Forces/1
  Magnetic Torques/1(Torque) -> Torques/1
  connections:
  brick reference/RConn1 -- Magnetic Torques/LConn1

== system tests/Subsystem/Single_Arm/Plate_2/Subsystem ==
  Slave_Moment : Inport
  Slave_Pos : Inport  Port=2
  Source_Moment : Inport  Port=3
  Source_Pos : Inport  Port=4
  Add : Sum  Inputs=+-
  Add1 : Sum  Inputs=+-
  Add2 : Sum  Inputs=+-
  Add3 : Sum  Inputs=+++
  Constant : Constant  Value=-3
  Constant1 : Constant  Value=-4
  Cross Product : matrix_library/Cross Product
  Dot Product : DotProduct  OutDataTypeStr=Inherit: Inherit via internal rule
  Dot Product1 : DotProduct  OutDataTypeStr=Inherit: Inherit via internal rule
  Gain : Gain  Gain=4*pi*1e-7/(4*pi)
  Gain1 : Gain  Gain=3
  Gain2 : Gain  Gain=3*4*pi*1e-7/(4*pi)
  Gain3 : Gain  Gain=5
  IdentityMatrix : IdentityMatrix  OutputDimensions=3
  Matrix Multiply : Product  Multiplication=Matrix(*)
  Matrix Multiply1 : Product  Multiplication=Matrix(*)
  Normalize Vector : vrlib/Utilities/Normalize Vector  maxzero=0
  Normalize Vector1 : vrlib/Utilities/Normalize Vector  maxzero=0
  Power : Math  Operator=pow
  Power1 : Math  Operator=pow
  Product{,1..5} (6 alike) : Product
  Sqrt : Sqrt
  Sqrt1 : Sqrt
  Transpose : Math  Operator=transpose
  m dot m : DotProduct  OutDataTypeStr=Inherit: Inherit via internal rule
  r dot m_master : DotProduct  OutDataTypeStr=Inherit: Inherit via internal rule
  r dot m_slave : DotProduct  OutDataTypeStr=Inherit: Inherit via internal rule
  Source_Torque : Outport
  Source_Force : Outport  Port=2
  wires:
  Power/1 -> Gain/1
  Transpose/1 -> Matrix Multiply/2
  Gain1/1 -> Add/1
  Matrix Multiply/1 -> Gain1/1
  Sqrt/1 -> Power/1
  Gain/1 -> Product/2
  Dot Product/1 -> Sqrt/1
  Product/1 -> Cross Product/2
  Matrix Multiply1/1 -> Product/1
  Normalize Vector/1 -> Transpose/1, Matrix Multiply/1
  IdentityMatrix/1 -> Add/2
  Constant/1 -> Power/2
  Add/1 -> Matrix Multiply1/1
  Slave_Pos/1 -> Add1/1
  Source_Pos/1 -> Add1/2
  Cross Product/1 -> Source_Torque/1
  Slave_Moment/1 -> Cross Product/1, Product2/2, m dot m/1, r dot m_slave/2
  Normalize Vector1/1 -> r dot m_slave/1, r dot m_master/1, Product4/2
  Add3/1 -> Product5/2
  Gain2/1 -> Product5/1
  Product4/1 -> Add3/3
  Dot Product1/1 -> Sqrt1/1
  Gain3/1 -> Add2/2
  r dot m_master/1 -> Product3/2, Product2/1
  Source_Moment/1 -> Matrix Multiply1/2, m dot m/2, Product1/2, r dot m_master/2
  m dot m/1 -> Add2/1
  Power1/1 -> Gain2/1
  Sqrt1/1 -> Power1/1
  r dot m_slave/1 -> Product1/1, Product3/1
  Product2/1 -> Add3/2
  Constant1/1 -> Power1/2
  Add2/1 -> Product4/1
  Add1/1 -> Normalize Vector1/1, Dot Product1/2, Dot Product1/1, Dot Product/2, Dot Product/1, Normalize Vector/1
  Product3/1 -> Gain3/1
  Product1/1 -> Add3/1
  Product5/1 -> Source_Force/1
